simulink model "Lokomat_Simulation"  (R2022b)
settings: Solver=FixedStepAuto  StartTime=0.0  StopTime=4  FixedStep=0.001  RelTol=1e-3
values from neighbouring files (symbols this model uses):
  kd = max(kd_hip)    [RMSE_code.m]    (also in Step_Hip.m = kd; Step_Knee.m = kd; Step_Response.m = max(kd_vec))
  kp = max(RMSE{length(kd_hip)}(:,1))    [RMSE_code.m]    (also in RMSE_hip.m = kp_vec_use(j); RMSE_knee.m = kp_vec_use(j); Step_Hip.m = kp; Step_Knee.m = kp)
undefined symbols (not defined in the file or in its folder): X, Y, Z
libraries: sm_lib x82, nesl_utility x9, simulink x6
(part 1 of 3)
Description:
  | load('Inputs.mat')
settings Model: Creator=mlnlab  LastModifiedBy=cster
settings DebuggingCC: UnconnectedInputMsg=warning  UnconnectedOutputMsg=warning  UnconnectedLineMsg=warning
settings ModelReferenceCC: EnableRefExpFcnMdlSchedulingChecks=on
settings RTWCC: DLArmComputeVersion=19.05

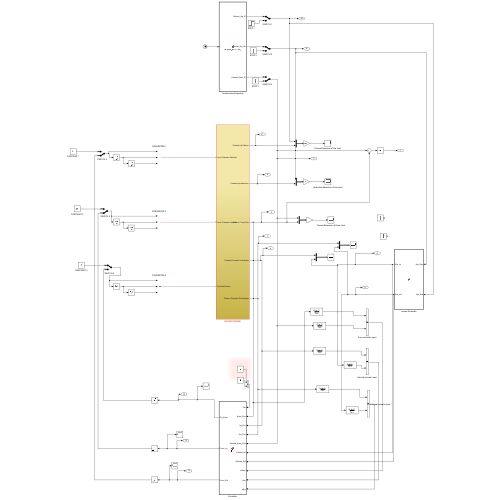
[thumbnail: Simulink's stored preview of the top-level diagram]
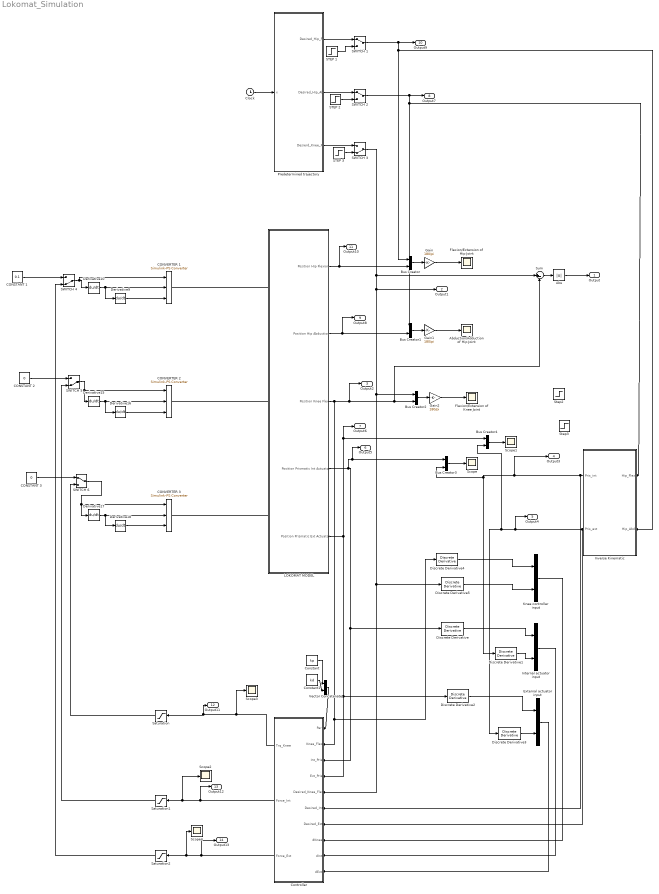
== system Lokomat_Simulation ==
  Abduction/Adduction of Hip Joint : Scope
  Abs : Abs  SaturateOnIntegerOverflow=off
  Bus Creator{,1..4} (5 alike) : BusCreator  Inputs=2
  CONSTANT 1 : Constant  Value=0.1
  CONSTANT 2 : Constant  Value=0
  CONSTANT 3 : Constant  Value=0
  CONVERTER 1 : nesl_utility/Simulink-PS Converter  PhysicalDomain=network_engine_domain  SubClassName=ps_input  LeftPortType=input  RightPortType=output  PseudoPeriodic=off  Frequencies=[]  NoiseDistribution=none  NoiseParameters=[]  Unit=N  AffineConversion=off  FilteringAndDerivatives=provide  SimscapeFilterOrder=1  InputFilterTimeConstant=0.001  UdotUserProvided=2
  "CONVERTER 2 " : nesl_utility/Simulink-PS Converter  PhysicalDomain=network_engine_domain  SubClassName=ps_input  LeftPortType=input  RightPortType=output  PseudoPeriodic=off  Frequencies=[]  NoiseDistribution=none  NoiseParameters=[]  Unit=N  AffineConversion=off  FilteringAndDerivatives=provide  SimscapeFilterOrder=1  InputFilterTimeConstant=0.001  UdotUserProvided=2
  CONVERTER 3 : nesl_utility/Simulink-PS Converter  PhysicalDomain=network_engine_domain  SubClassName=ps_input  LeftPortType=input  RightPortType=output  PseudoPeriodic=off  Frequencies=[]  NoiseDistribution=none  NoiseParameters=[]  Unit=rad  AffineConversion=off  FilteringAndDerivatives=provide  SimscapeFilterOrder=1  InputFilterTimeConstant=0.001  UdotUserProvided=2
  Clock : Clock
  Constant : Constant  Value=kp
  Constant1 : Constant  Value=kd
  "Controller " : MATLAB Function  TreatAsAtomicUnit=on
  Derivative{9..10,15..18} (6 alike) : Derivative
  Discrete Derivative{,1..5} (6 alike) : simulink/Quick Insert/Discrete/Discrete Derivative  gainval=1.0  ICPrevScaledInput=0.0  OutMin=[]  OutMax=[]  OutDataType=fixdt(1, 16)  OutScaling=2^-10  DoSatur=off
  External actuator input : Concatenate
  Flexion/Extension of Hip Joint : Scope
  Flexion/Extension of Knee Joint : Scope
  Gain : Gain  Gain=180/pi
  Gain1 : Gain  Gain=180/pi
  Gain2 : Gain  Gain=180/pi
  Internal actuator input : Concatenate
  "Inverse Kinematic " : MATLAB Function  TreatAsAtomicUnit=on
  Knee controller input : Concatenate
  LOKOMAT MODEL : Subsystem
  Predetermined trajectory : MATLAB Function  TreatAsAtomicUnit=on
  STEP 1 : Step  Time=2  After=(0.5/180)*3.14159*0  SampleTime=0
  STEP 2 : Step  Time=2  After=(0.5/180)*3.14159*0  SampleTime=0
  STEP 3 : Step  Time=2  After=-(1/180)*3.14159*0  SampleTime=0
  SWITCH 1 : ManualSwitch
  SWITCH 2 : ManualSwitch
  SWITCH 3 : ManualSwitch  CurrentSetting=0
  SWITCH 4 : ManualSwitch  CurrentSetting=0
  SWITCH 5 : ManualSwitch  CurrentSetting=0
  SWITCH 6 : ManualSwitch
  Saturation : Saturate  UpperLimit=20  LowerLimit=-20
  Saturation1 : Saturate  UpperLimit=500  LowerLimit=-500
  Saturation2 : Saturate  UpperLimit=500  LowerLimit=-500
  Scope{,1..4} (5 alike) : Scope
  Step2 : Step  After=0.01  SampleTime=0
  Step3 : Step  After=0.01  SampleTime=0
  Sum : Sum  Inputs=|+-
  Vector Concatenate : Concatenate
  Output : Outport
  Output1 : Outport  Port=2
  Output2 : Outport  Port=3
  Output3 : Outport  Port=4
  Output4 : Outport  Port=5
  Output5 : Outport  Port=6
  Output6 : Outport  Port=7
  Output7 : Outport  Port=8
  Output8 : Outport  Port=9
  Output9 : Outport  Port=10
  Output10 : Outport  Port=11
  Output11 : Outport  Port=12
  Output12 : Outport  Port=13
  Output13 : Outport  Port=14
  wires:
  Bus Creator/1 -> Gain/1
  Bus Creator1/1 -> Gain1/1
  Gain/1 -> Flexion/Extension of Hip Joint/1
  Gain1/1 -> Abduction/Adduction of Hip Joint/1
  Derivative10/1 -> Derivative9/1, CONVERTER 1/2
  Derivative15/1 -> "CONVERTER 2 "/2, Derivative16/1
  Derivative17/1 -> Derivative18/1, CONVERTER 3/2
  Derivative16/1 -> "CONVERTER 2 "/3
  Derivative9/1 -> CONVERTER 1/3
  Derivative18/1 -> CONVERTER 3/3
  LOKOMAT MODEL/1(Position Hip Flexion) -> Output10/1, Bus Creator/2
  LOKOMAT MODEL/2(Position Hip Abduction) -> Output8/1, Bus Creator1/2
  Clock/1 -> Predetermined trajectory/1(x)
  LOKOMAT MODEL/3(Position Knee Flex) -> Output2/1, Bus Creator2/2, Sum/2, Discrete Derivative4/1, "Controller "/2(Knee_Flex)
  Gain2/1 -> Flexion/Extension of Knee Joint/1
  Bus Creator2/1 -> Gain2/1
  SWITCH 3/1 -> Output1/1, Bus Creator2/1, "Controller "/5(Desired_Knee_Flex), Discrete Derivative5/1, Sum/1
  Discrete Derivative4/1 -> Knee controller input/1
  Discrete Derivative5/1 -> Knee controller input/2
  Knee controller input/1 -> "Controller "/8(dKnee)
  "Inverse Kinematic "/1(Pris_int) -> Output3/1, Discrete Derivative1/1, Bus Creator3/2, "Controller "/6(Desired_Int)
  LOKOMAT MODEL/4(Position Prismatic Int Actuator) -> Discrete Derivative/1, "Controller "/3(Int_Pris), Output5/1, Bus Creator3/1
  LOKOMAT MODEL/5(Position Prismatic Ext Actuator) -> Output6/1, Bus Creator4/1, "Controller "/4(Ext_Pris), Discrete Derivative2/1
  "Inverse Kinematic "/2(Pris_ext) -> "Controller "/7(Desired_Ext), Discrete Derivative3/1, Bus Creator4/2, Output4/1
  Internal actuator input/1 -> "Controller "/9(dInt)
  External actuator input/1 -> "Controller "/10(dExt)
  Bus Creator3/1 -> Scope/1
  Bus Creator4/1 -> Scope1/1
  Sum/1 -> Abs/1
  Abs/1 -> Output/1
  Constant1/1 -> Vector Concatenate/2
  Constant/1 -> Vector Concatenate/1
  Vector Concatenate/1 -> "Controller "/1(Par)
  "Controller "/1(Trq_Knee) -> Scope3/1, Output11/1, Saturation/1
  SWITCH 1/1 -> Output9/1, Bus Creator/1, "Inverse Kinematic "/2(Hip_Abd)
  Discrete Derivative/1 -> Internal actuator input/1
  Discrete Derivative1/1 -> Internal actuator input/2
  Discrete Derivative2/1 -> External actuator input/1
  Discrete Derivative3/1 -> External actuator input/2
  "Controller "/2(Force_Int) -> Output12/1, Scope2/1, Saturation1/1
  "Controller "/3(Force_Ext) -> Output13/1, Scope4/1, Saturation2/1
  CONSTANT 3/1 -> SWITCH 6/1
  CONSTANT 2/1 -> SWITCH 5/1
  CONSTANT 1/1 -> SWITCH 4/1
  SWITCH 4/1 -> CONVERTER 1/1, Derivative10/1
  Saturation2/1 -> SWITCH 4/2
  SWITCH 5/1 -> "CONVERTER 2 "/1, Derivative15/1
  Saturation1/1 -> SWITCH 5/2
  SWITCH 6/1 -> CONVERTER 3/1, Derivative17/1
  Saturation/1 -> SWITCH 6/2
  Predetermined trajectory/3(Desierd_Knee_Fl) -> SWITCH 3/1
  STEP 3/1 -> SWITCH 3/2
  STEP 2/1 -> SWITCH 2/2
  Predetermined trajectory/2(Desired_Hip_Ab) -> SWITCH 2/1
  STEP 1/1 -> SWITCH 1/2
  Predetermined trajectory/1(Desired_Hip_Fl) -> SWITCH 1/1
  SWITCH 2/1 -> Output7/1, Bus Creator1/1, "Inverse Kinematic "/1(Hip_Flex)
  connections:
  LOKOMAT MODEL/LConn3 -- CONVERTER 3/RConn1
  LOKOMAT MODEL/LConn2 -- "CONVERTER 2 "/RConn1
  LOKOMAT MODEL/LConn1 -- CONVERTER 1/RConn1
